simulink model "IID_nms_2Dmodel_for"  (R2016b)
settings: Solver=ode15s  StartTime=0.0  StopTime=t_end  FixedStep=1e-3  MaxStep=ts_max  RelTol=1e-3  AbsTol=1e-4  EnableMultiTasking=on
InitFcn:
  | IID_runScripts;
values from neighbouring files (symbols this model uses):
  D12_F = 0.16    [IID_nms_MechInit.m]    (also in nms_MechInit.m)
  D12_S = L_S    (= 0.5)    [IID_nms_MechInit.m]    (also in nms_MechInit.m = 0.46)
  D12_T = L_T    (= 0.5)    [IID_nms_MechInit.m]    (also in nms_MechInit.m = 0.46)
  D13_F = 0.20    (= 0.2)    [IID_nms_MechInit.m]    (also in nms_MechInit.m)
  D1G_F = 0.14    [IID_nms_MechInit.m]    (also in nms_MechInit.m)
  D1G_HAT = 0.35    [IID_nms_MechInit.m]    (also in nms_MechInit.m)
  D1G_S = 0.3    [IID_nms_MechInit.m]    (also in nms_MechInit.m = 0.28)
  D1G_T = 0.3    [IID_nms_MechInit.m]    (also in nms_MechInit.m = 0.28)
  DeltaThRef = 5e-3    (= 0.005)    [IID_nms_MechInit.m]    (also in nms_MechInit.m)
  Dist_On = 1    [IID_setDistPar.m]    (also in setDistPar.m)
  Dist_PDur = 0.15    [IID_setDistPar.m]    (also in setDistPar.m)
  Dist_StartTime = 15    [IID_setDistPar.m]    (also in setDistPar.m)
  Dist_xyzHAT_sag_PH = 0    [IID_setDistPar.m]    (also in setDistPar.m)
  In_F = 0.005    [IID_nms_MechInit.m]    (also in nms_MechInit.m)
  In_HAT = 3    [IID_nms_MechInit.m]    (also in nms_MechInit.m = 2.5)
  In_S = 0.05    [IID_nms_MechInit.m]    (also in nms_MechInit.m)
  In_T = 0.15    [IID_nms_MechInit.m]    (also in nms_MechInit.m)
  k_gx = (2*(m_F+m_S+m_T)+m_HAT)*g/0.1    (= 7848)    [IID_nms_MechInit.m]
  k_gy = (2*(m_F+m_S+m_T)+m_HAT)*g/0.01    (= 78480)    [IID_nms_MechInit.m]
  k_pressure = m_HAT * 9.81 / DeltaThRef    (= 104967)    [IID_nms_MechInit.m]    (also in nms_MechInit.m)
  m_F = 1.25    [IID_nms_MechInit.m]    (also in nms_MechInit.m)
  m_HAT = 53.5    [IID_nms_MechInit.m]    (also in nms_MechInit.m)
  m_S = 3.5    [IID_nms_MechInit.m]    (also in nms_MechInit.m)
  m_T = 8.5    [IID_nms_MechInit.m]    (also in nms_MechInit.m)
  m_Total = m_F*2+m_S*2+m_T*2+m_HAT    (= 80)    [IID_nms_MechInit.m]    (also in nms_MechInit.m)
  MidDelay = 0.010    (= 0.01)    [IID_setCtrlPar.m]    (also in nms_MechInit.m = 0.005)
  mu_slide = 0.8    [IID_nms_MechInit.m]    (also in nms_MechInit.m)
  mu_stick = 0.9    [IID_nms_MechInit.m]    (also in nms_MechInit.m)
  N = 1.5    [IID_nms_MechInit.m]    (also in cmaes_parfor.m = size(x,1); nms_MechInit.m)
  s = x(1:N-1,:).^2 + x(2:N,:).^2    [cmaes_parfor.m]
  ThPos = 4/5    (= 0.8)    [IID_nms_MechInit.m]    (also in nms_MechInit.m)
  v_gx_max = 0.03    [IID_nms_MechInit.m]
  v_gy_max = 0.03    [IID_nms_MechInit.m]
  v_max_pressure = 0.5    [IID_nms_MechInit.m]    (also in nms_MechInit.m)
  vLimit = 0.01    [IID_nms_MechInit.m]    (also in nms_MechInit.m)
undefined symbols (not defined in the file or in its folder): sgn
libraries: mblibv1 x71, cpg_lib x23, simulink x21, simulink_extras x6
(part 2 of 3)

== system IID_nms_2Dmodel_for/Signals NMC Left7 ==
  Mux : Mux  Inputs=7
  signals : Outport
  wires:
  Mux/1 -> signals/1
  [LEnergyVAS] -> Mux/2
  [LEnergyHFL] -> Mux/1
  [LEnergyTA] -> Mux/3
  [LEnergySOL] -> Mux/4
  [LEnergyHAM] -> Mux/6
  [LEnergyGAS] -> Mux/5
  [LEnergyGLU] -> Mux/7

== system IID_nms_2Dmodel_for/Signals NMC Right3 ==
  Mux : Mux
  signals : Outport
  wires:
  Mux/1 -> signals/1
  [RM34] -> Mux/1
  [RM23] -> Mux/3
  [RM12] -> Mux/4
  [RM34R] -> Mux/2

== system IID_nms_2Dmodel_for/etc ==
  note: Fall detection
      | (stop simulation)
  Abs3 : Abs
  Compare To Constant2 : simulink/Logic and Bit Operations/Compare To Constant  relop=>  const=60*pi/180  OutDataTypeStr=boolean
  Stop Simulation : Stop
  wires:
  Compare To Constant2/1 -> Stop Simulation/1
  Abs3/1 -> Compare To Constant2/1
  [theta] -> Abs3/1

== system IID_nms_2Dmodel_for/Body Mechanics Layer/Left Force Plate ==
  "GRF_Ball [N N] " : Inport
  GRF_Heel [N N] : Inport  Port=2
  Enable : EnablePort  StatesWhenEnabling=reset
  Fcn : Fcn  Expr=u(1)/(u(2)+eps)
  Mux : Mux  Inputs=3
  Mux1 : Mux  Inputs=2
  Selector : Selector  InputPortWidth=2  IndexOptions=Index vector (dialog)  Indices=2  OutputSizes=1
  Selector1 : Selector  InputPortWidth=2  IndexOptions=Index vector (dialog)  Indices=2  OutputSizes=1
  Sum1 : Sum
  GRFs : Outport  OutputWhenDisabled=reset  InitialOutput=0
  COP : Outport  Port=2  OutputWhenDisabled=reset  InitialOutput=0
  wires:
  Selector/1 -> Mux1/2
  Selector1/1 -> Mux1/1
  "GRF_Ball [N N] "/1 -> Sum1/1, Mux/1, Selector1/1
  GRF_Heel [N N]/1 -> Sum1/2, Mux/3
  Sum1/1 -> Mux/2, Selector/1
  Mux/1 -> GRFs/1
  Mux1/1 -> Fcn/1
  Fcn/1 -> COP/1

== system IID_nms_2Dmodel_for/Body Mechanics Layer/Left Leg Load ==
  dxThigh [m] : Inport
  FB Gain1 : Gain  Gain=1/DeltaThRef  SaturateOnIntegerOverflow=on  OutDataTypeStr=Inherit: Same as input  ParamDataTypeStr=Inherit: Same as input
  Saturation11 : Saturate  UpperLimit=inf  LowerLimit=0  ZeroCross=off
  smooth2 : TransferFcn  Denominator=[0.02 1]
  LLoad [F] : Outport
  wires:
  dxThigh [m]/1 -> smooth2/1
  FB Gain1/1 -> LLoad [F]/1
  smooth2/1 -> Saturation11/1
  Saturation11/1 -> FB Gain1/1

== system IID_nms_2Dmodel_for/Body Mechanics Layer/Left Thigh Sensor Sheet ==
  note: Inner Segment Pressure Sheet
  Gain3 : Gain  Gain=k_pressure
  Gain4 : Gain  Gain=1/v_max_pressure
  Inner Thigh Shift Joint : mblibv1/Joints/Prismatic  LConnTagsString=__newl0|SA1|SA2  RConnTagsString=__newr0|SA1  UpdateFromCAD=off  NumSAPorts=3  CutJoint=off  MarkAsCut=off  Primitives=prismatic  PrimitiveProps=P1$WORLD$[1 0 0]$prismatic  DialogClass=JointBlock  P1Axis=[1 0 0]
  Left Thigh Sensor Sheet IC : mblibv1/Sensors &  Actuators/Joint Initial Condition  UpdateFromCAD=off  LeftPortType=blob  RightPortType=blob  PhysicalDomain=mechanical  DialogClass=InitialConditionBlock  InitialConditions=P1$true$0$m$rad$0$m/s$rad/s#P2$false$0$m$rad$0$m/s$rad/s#P3$false$0$m$rad$0$m/s$rad/s#R1$false$0$m$rad$0$m/s$rad/s#R2$false$0$m$rad$0$m/s$rad/s#R3$false$0$m$rad$0$m/s$rad/s#S$false$0$m$rad$0$m/s$rad/s  P1PIC=0  P1VIC=0  P2PIC=0  P2VIC=0  P3PIC=0  P3VIC=0  R1PIC=0  R1VIC=0  R2PIC=0  R2VIC=0  R3PIC=0  R3VIC=0  SPIC=0  SVIC=0
  Mux1 : Mux  Inputs=2
  Pressure Sheet Reaction Force : Fcn  Expr=-u(1) * (1+sgn(u(1))*u(2))
  Thigh Actuator : mblibv1/Sensors &  Actuators/Joint Actuator  UpdateFromCAD=off  PhysicalDomain=Mechanical  PortType=blob  ActuationStyle=Force  AngleUnits=deg  ArcVelocityUnits=deg/s  ArcAccelerationUnits=deg/s^2  CoordPositionUnits=m  VelocityUnits=m/s  AccelerationUnits=m/s^2  ForceUnits=N  TorqueUnits=N-m  ActiveIO=on  Width=1  DialogClass=MechanicalActuatorBlock  Primitive=P1  ReferenceFrame=Absolute (INERTIAL)
  Thigh Sensor : mblibv1/Sensors &  Actuators/Joint Sensor  UpdateFromCAD=off  PhysicalDomain=Mechanical  PortType=blob  Muxed=off  Pose=off  Angle=on  AngleUnits=deg  ArcVelocity=off  ArcVelocityUnits=deg/s  ArcAcceleration=off  ArcAccelerationUnits=deg/s^2  CoordPosition=on  CoordPositionUnits=m  Velocity=on  VelocityUnits=m/s  Acceleration=off  AccelerationUnits=m/s^2  Quaternion=on  QuaternionDT=off  QuaternionDDT=off  QuaternionUnits=off  OutputVector=[ 1 1 ]  ActiveIO=on  Width=2  DialogClass=MechanicalSensorBlock  Primitive=P1  Force=off  ForceUnits=N  Torque=off  TorqueUnits=N-m  ReferenceFrame=Absolute (INERTIAL)  ReactionSensedSide=Base  ReactionReferenceFrame=Absolute (World)  ReactionForce=off  ReactionForceUnits=N  ReactionMoment=off  ReactionMomentUnits=N-m
  B : PMIOPort  Tag=PMCPort  Port=1  Side=Left
  F : PMIOPort  Tag=PMCPort  Port=2  Side=Right
  dx : Outport
  wires:
  Thigh Sensor/1 -> Gain3/1, dx/1
  Thigh Sensor/2 -> Gain4/1
  Mux1/1 -> Pressure Sheet Reaction Force/1
  Gain3/1 -> Mux1/1
  Gain4/1 -> Mux1/2
  Pressure Sheet Reaction Force/1 -> Thigh Actuator/1
  connections:
  B/RConn1 -- Inner Thigh Shift Joint/LConn1
  F/RConn1 -- Inner Thigh Shift Joint/RConn1
  Thigh Sensor/LConn1 -- Inner Thigh Shift Joint/LConn2
  Inner Thigh Shift Joint/RConn2 -- Thigh Actuator/RConn1
  Left Thigh Sensor Sheet IC/RConn1 -- Inner Thigh Shift Joint/LConn3

== system IID_nms_2Dmodel_for/Body Mechanics Layer/RLBall Cnt1 ==
  note: 3D Ground Interaction Model
  Dist_sag : Inport
  Body Actuator : mblibv1/Sensors &  Actuators/Body Actuator  UpdateFromCAD=off  PhysicalDomain=Mechanical  PortType=blob  ActuationStyle=Force  AngleUnits=deg  ArcVelocityUnits=deg/s  ArcAccelerationUnits=deg/s^2  CoordPositionUnits=m  VelocityUnits=m/s  AccelerationUnits=m/s^2  ForceUnits=N  TorqueUnits=N*m  ActiveIO=on  Width=3  DialogClass=MechanicalActuatorBlock  ReferenceFrame=Local (Body CS)  Angle=off  CoordPosition=on  Force=on  Torque=off
  Constant : Constant  Value=0
  Gain : Gain  Gain=-1
  Mechanical Branching Bar : mblibv1/Utilities/Mechanical Branching Bar  LConnTagsString=_newl0  RConnTagsString=SA0|SA1  UpdateFromCAD=off  DialogClass=MechanicalBranchingBarBlock  NumSAPorts=2
  Mux : Mux  Inputs=3
  Product : Product
  Product1 : Product
  Right Heel Sensor5 : mblibv1/Sensors &  Actuators/Body Sensor  UpdateFromCAD=off  PhysicalDomain=Mechanical  PortType=blob  Muxed=off  Pose=on  Angle=on  AngleUnits=deg  ArcVelocity=off  ArcVelocityUnits=deg/s  ArcAcceleration=off  ArcAccelerationUnits=deg/s^2  CoordPosition=on  CoordPositionUnits=m  Velocity=off  VelocityUnits=m/s  Acceleration=off  AccelerationUnits=m/s^2  Quaternion=on  QuaternionDT=off  QuaternionDDT=off  QuaternionUnits=off  OutputVector=[ 3 3 ]  ActiveIO=on  Width=12  DialogClass=MechanicalSensorBlock  ReferenceFrame=Absolute (World)
  Trigonometric Function : Trigonometry  Operator=cos
  Trigonometric Function1 : Trigonometry
  F : PMIOPort  Port=1  Side=Left
  Pos : Outport
  Rot : Outport  Port=2
  wires:
  Right Heel Sensor5/1 -> Pos/1  "pos"
  Mux/1 -> Body Actuator/1
  Constant/1 -> Mux/3
  Right Heel Sensor5/2 -> Rot/1
  [theta] -> Trigonometric Function/1, Trigonometric Function1/1
  Dist_sag/1 -> Product1/2, Product/2
  Trigonometric Function/1 -> Product/1
  Product/1 -> Gain/1
  Gain/1 -> Mux/2
  Trigonometric Function1/1 -> Product1/1
  Product1/1 -> Mux/1
  connections:
  F/RConn1 -- Mechanical Branching Bar/LConn1
  Mechanical Branching Bar/RConn2 -- Body Actuator/RConn1
  Mechanical Branching Bar/RConn1 -- Right Heel Sensor5/LConn1

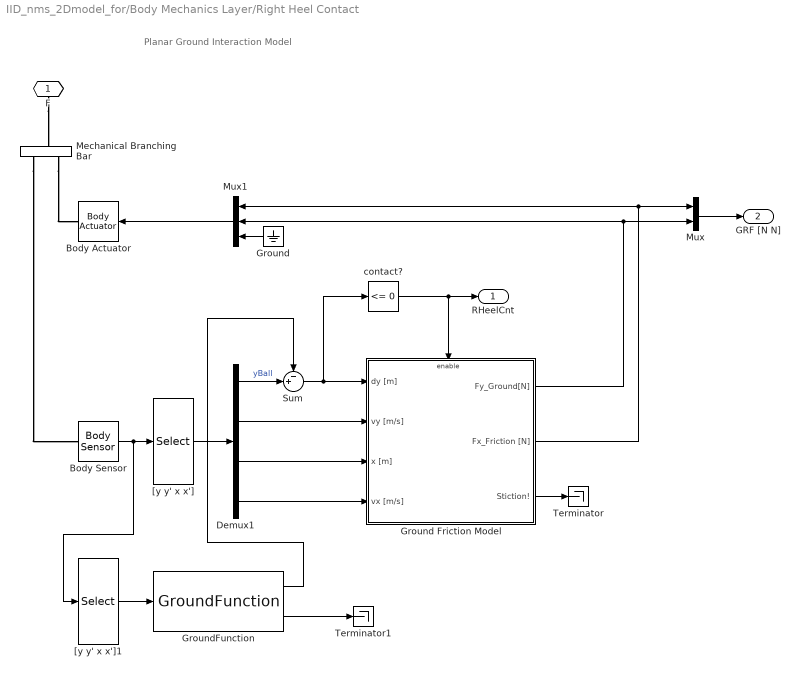
== system IID_nms_2Dmodel_for/Body Mechanics Layer/Right Heel Contact ==
  note: Planar Ground Interaction Model
  Body Actuator : mblibv1/Sensors &  Actuators/Body Actuator  UpdateFromCAD=off  PhysicalDomain=Mechanical  PortType=blob  ActuationStyle=Force  AngleUnits=deg  ArcVelocityUnits=deg/s  ArcAccelerationUnits=deg/s^2  CoordPositionUnits=m  VelocityUnits=m/s  AccelerationUnits=m/s^2  ForceUnits=N  TorqueUnits=N-m  ActiveIO=on  Width=3  DialogClass=MechanicalActuatorBlock  ReferenceFrame=Absolute (World)  Angle=off  CoordPosition=on  Force=on  Torque=off
  Body Sensor : mblibv1/Sensors &  Actuators/Body Sensor  UpdateFromCAD=off  PhysicalDomain=Mechanical  PortType=blob  Muxed=on  Pose=off  Angle=on  AngleUnits=deg  ArcVelocity=off  ArcVelocityUnits=deg/s  ArcAcceleration=off  ArcAccelerationUnits=deg/s^2  CoordPosition=on  CoordPositionUnits=m  Velocity=on  VelocityUnits=m/s  Acceleration=off  AccelerationUnits=m/s^2  Quaternion=on  QuaternionDT=off  QuaternionDDT=off  QuaternionUnits=off  OutputVector=[ 3 3 ]  ActiveIO=on  Width=6  DialogClass=MechanicalSensorBlock  ReferenceFrame=Absolute (World)
  Demux1 : Demux
  Ground : Ground
  Ground Friction Model : Subsystem
  GroundFunction : cpg_lib/GroundFunction
  Mechanical Branching Bar : mblibv1/Utilities/Mechanical Branching Bar  LConnTagsString=_newl0  RConnTagsString=SA0|SA1  UpdateFromCAD=off  DialogClass=MechanicalBranchingBarBlock  NumSAPorts=2
  Mux : Mux  Inputs=2
  Mux1 : Mux  Inputs=3
  Sum : Sum  Inputs=-+|
  Terminator : Terminator
  Terminator1 : Terminator
  "[y y' x x']" : Selector  InputPortWidth=6  IndexOptions=Index vector (dialog)  Indices=[2 5 1 4]  OutputSizes=1
  "[y y' x x']1" : Selector  InputPortWidth=6  IndexOptions=Index vector (dialog)  Indices=[1 2 3]  OutputSizes=1
  contact? : simulink/Logic and Bit Operations/Compare To Zero  relop=<=  OutDataTypeStr=boolean
  F : PMIOPort  Port=1  Side=Left
  RHeelCnt : Outport
  GRF [N N] : Outport  Port=2
  wires:
  Ground Friction Model/3(Stiction!) -> Terminator/1
  Ground Friction Model/2(Fx_Friction [N]) -> Mux/1, Mux1/1
  Ground Friction Model/1(Fy_Ground[N]) -> Mux/2, Mux1/2
  contact?/1 -> Ground Friction Model/Enable, RHeelCnt/1
  Demux1/4 -> Ground Friction Model/4(vx [m/s])
  Demux1/3 -> Ground Friction Model/3(x [m])
  Demux1/2 -> Ground Friction Model/2(vy [m/s])
  Mux/1 -> GRF [N N]/1
  GroundFunction/1 -> Sum/1
  Demux1/1 -> Sum/2  "yBall"
  Sum/1 -> Ground Friction Model/1(dy [m]), contact?/1
  Body Sensor/1 -> "[y y' x x']1"/1, "[y y' x x']"/1
  "[y y' x x']"/1 -> Demux1/1
  Mux1/1 -> Body Actuator/1
  Ground/1 -> Mux1/3
  "[y y' x x']1"/1 -> GroundFunction/1
  GroundFunction/2 -> Terminator1/1
  connections:
  F/RConn1 -- Mechanical Branching Bar/LConn1
  Mechanical Branching Bar/RConn1 -- Body Sensor/LConn1
  Mechanical Branching Bar/RConn2 -- Body Actuator/RConn1

== system IID_nms_2Dmodel_for/Body Mechanics Layer/Right Heel Contact1 ==
  note: Planar Ground Interaction Model
  Body Actuator : mblibv1/Sensors &  Actuators/Body Actuator  UpdateFromCAD=off  PhysicalDomain=Mechanical  PortType=blob  ActuationStyle=Force  AngleUnits=deg  ArcVelocityUnits=deg/s  ArcAccelerationUnits=deg/s^2  CoordPositionUnits=m  VelocityUnits=m/s  AccelerationUnits=m/s^2  ForceUnits=N  TorqueUnits=N-m  ActiveIO=on  Width=3  DialogClass=MechanicalActuatorBlock  ReferenceFrame=Absolute (World)  Angle=off  CoordPosition=on  Force=on  Torque=off
  Body Sensor : mblibv1/Sensors &  Actuators/Body Sensor  UpdateFromCAD=off  PhysicalDomain=Mechanical  PortType=blob  Muxed=on  Pose=off  Angle=on  AngleUnits=deg  ArcVelocity=off  ArcVelocityUnits=deg/s  ArcAcceleration=off  ArcAccelerationUnits=deg/s^2  CoordPosition=on  CoordPositionUnits=m  Velocity=on  VelocityUnits=m/s  Acceleration=off  AccelerationUnits=m/s^2  Quaternion=on  QuaternionDT=off  QuaternionDDT=off  QuaternionUnits=off  OutputVector=[ 3 3 ]  ActiveIO=on  Width=6  DialogClass=MechanicalSensorBlock  ReferenceFrame=Absolute (World)
  Demux1 : Demux
  Ground : Ground
  Ground Friction Model : Subsystem
  GroundFunction : cpg_lib/GroundFunction
  Mechanical Branching Bar : mblibv1/Utilities/Mechanical Branching Bar  LConnTagsString=_newl0  RConnTagsString=SA0|SA1  UpdateFromCAD=off  DialogClass=MechanicalBranchingBarBlock  NumSAPorts=2
  Mux : Mux  Inputs=2
  Mux1 : Mux  Inputs=3
  Sum : Sum  Inputs=-+|
  Terminator : Terminator
  Terminator1 : Terminator
  "[y y' x x']" : Selector  InputPortWidth=6  IndexOptions=Index vector (dialog)  Indices=[2 5 1 4]  OutputSizes=1
  "[y y' x x']1" : Selector  InputPortWidth=6  IndexOptions=Index vector (dialog)  Indices=[1 2 3]  OutputSizes=1
  contact? : simulink/Logic and Bit Operations/Compare To Zero  relop=<=  OutDataTypeStr=boolean
  F : PMIOPort  Port=1  Side=Left
  RHeelCnt : Outport
  GRF [N N] : Outport  Port=2
  wires:
  GroundFunction/2 -> Terminator1/1
  "[y y' x x']1"/1 -> GroundFunction/1
  Ground/1 -> Mux1/3
  Mux1/1 -> Body Actuator/1
  "[y y' x x']"/1 -> Demux1/1
  Body Sensor/1 -> "[y y' x x']"/1, "[y y' x x']1"/1
  Sum/1 -> contact?/1, Ground Friction Model/1(dy [m])
  Demux1/1 -> Sum/2  "yBall"
  GroundFunction/1 -> Sum/1
  Mux/1 -> GRF [N N]/1
  Demux1/2 -> Ground Friction Model/2(vy [m/s])
  Demux1/3 -> Ground Friction Model/3(x [m])
  Demux1/4 -> Ground Friction Model/4(vx [m/s])
  contact?/1 -> RHeelCnt/1, Ground Friction Model/Enable
  Ground Friction Model/1(Fy_Ground[N]) -> Mux1/2, Mux/2
  Ground Friction Model/2(Fx_Friction [N]) -> Mux1/1, Mux/1
  Ground Friction Model/3(Stiction!) -> Terminator/1
  connections:
  Mechanical Branching Bar/RConn2 -- Body Actuator/RConn1
  Mechanical Branching Bar/RConn1 -- Body Sensor/LConn1
  F/RConn1 -- Mechanical Branching Bar/LConn1

== system IID_nms_2Dmodel_for/Body Mechanics Layer/Right Heel Contact2 ==
  note: Planar Ground Interaction Model
  Body Actuator : mblibv1/Sensors &  Actuators/Body Actuator  UpdateFromCAD=off  PhysicalDomain=Mechanical  PortType=blob  ActuationStyle=Force  AngleUnits=deg  ArcVelocityUnits=deg/s  ArcAccelerationUnits=deg/s^2  CoordPositionUnits=m  VelocityUnits=m/s  AccelerationUnits=m/s^2  ForceUnits=N  TorqueUnits=N-m  ActiveIO=on  Width=3  DialogClass=MechanicalActuatorBlock  ReferenceFrame=Absolute (World)  Angle=off  CoordPosition=on  Force=on  Torque=off
  Body Sensor : mblibv1/Sensors &  Actuators/Body Sensor  UpdateFromCAD=off  PhysicalDomain=Mechanical  PortType=blob  Muxed=on  Pose=off  Angle=on  AngleUnits=deg  ArcVelocity=off  ArcVelocityUnits=deg/s  ArcAcceleration=off  ArcAccelerationUnits=deg/s^2  CoordPosition=on  CoordPositionUnits=m  Velocity=on  VelocityUnits=m/s  Acceleration=off  AccelerationUnits=m/s^2  Quaternion=on  QuaternionDT=off  QuaternionDDT=off  QuaternionUnits=off  OutputVector=[ 3 3 ]  ActiveIO=on  Width=6  DialogClass=MechanicalSensorBlock  ReferenceFrame=Absolute (World)
  Demux1 : Demux
  Ground : Ground
  Ground Friction Model : Subsystem
  GroundFunction : cpg_lib/GroundFunction
  Mechanical Branching Bar : mblibv1/Utilities/Mechanical Branching Bar  LConnTagsString=_newl0  RConnTagsString=SA0|SA1  UpdateFromCAD=off  DialogClass=MechanicalBranchingBarBlock  NumSAPorts=2
  Mux : Mux  Inputs=2
  Mux1 : Mux  Inputs=3
  Sum : Sum  Inputs=-+|
  Terminator : Terminator
  Terminator1 : Terminator
  "[y y' x x']" : Selector  InputPortWidth=6  IndexOptions=Index vector (dialog)  Indices=[2 5 1 4]  OutputSizes=1
  "[y y' x x']1" : Selector  InputPortWidth=6  IndexOptions=Index vector (dialog)  Indices=[1 2 3]  OutputSizes=1
  contact? : simulink/Logic and Bit Operations/Compare To Zero  relop=<=  OutDataTypeStr=boolean
  F : PMIOPort  Port=1  Side=Left
  RHeelCnt : Outport
  GRF [N N] : Outport  Port=2
  wires:
  Ground Friction Model/3(Stiction!) -> Terminator/1
  Ground Friction Model/2(Fx_Friction [N]) -> Mux/1, Mux1/1
  Ground Friction Model/1(Fy_Ground[N]) -> Mux/2, Mux1/2
  contact?/1 -> Ground Friction Model/Enable, RHeelCnt/1
  Demux1/4 -> Ground Friction Model/4(vx [m/s])
  Demux1/3 -> Ground Friction Model/3(x [m])
  Demux1/2 -> Ground Friction Model/2(vy [m/s])
  Mux/1 -> GRF [N N]/1
  GroundFunction/1 -> Sum/1
  Demux1/1 -> Sum/2  "yBall"
  Sum/1 -> Ground Friction Model/1(dy [m]), contact?/1
  Body Sensor/1 -> "[y y' x x']1"/1, "[y y' x x']"/1
  "[y y' x x']"/1 -> Demux1/1
  Mux1/1 -> Body Actuator/1
  Ground/1 -> Mux1/3
  "[y y' x x']1"/1 -> GroundFunction/1
  GroundFunction/2 -> Terminator1/1
  connections:
  F/RConn1 -- Mechanical Branching Bar/LConn1
  Mechanical Branching Bar/RConn1 -- Body Sensor/LConn1
  Mechanical Branching Bar/RConn2 -- Body Actuator/RConn1

== system IID_nms_2Dmodel_for/Body Mechanics Layer/Right Heel Contact3 ==
  note: Planar Ground Interaction Model
  Body Actuator : mblibv1/Sensors &  Actuators/Body Actuator  UpdateFromCAD=off  PhysicalDomain=Mechanical  PortType=blob  ActuationStyle=Force  AngleUnits=deg  ArcVelocityUnits=deg/s  ArcAccelerationUnits=deg/s^2  CoordPositionUnits=m  VelocityUnits=m/s  AccelerationUnits=m/s^2  ForceUnits=N  TorqueUnits=N-m  ActiveIO=on  Width=3  DialogClass=MechanicalActuatorBlock  ReferenceFrame=Absolute (World)  Angle=off  CoordPosition=on  Force=on  Torque=off
  Body Sensor : mblibv1/Sensors &  Actuators/Body Sensor  UpdateFromCAD=off  PhysicalDomain=Mechanical  PortType=blob  Muxed=on  Pose=off  Angle=on  AngleUnits=deg  ArcVelocity=off  ArcVelocityUnits=deg/s  ArcAcceleration=off  ArcAccelerationUnits=deg/s^2  CoordPosition=on  CoordPositionUnits=m  Velocity=on  VelocityUnits=m/s  Acceleration=off  AccelerationUnits=m/s^2  Quaternion=on  QuaternionDT=off  QuaternionDDT=off  QuaternionUnits=off  OutputVector=[ 3 3 ]  ActiveIO=on  Width=6  DialogClass=MechanicalSensorBlock  ReferenceFrame=Absolute (World)
  Demux1 : Demux
  Ground : Ground
  Ground Friction Model : Subsystem
  GroundFunction : cpg_lib/GroundFunction
  Mechanical Branching Bar : mblibv1/Utilities/Mechanical Branching Bar  LConnTagsString=_newl0  RConnTagsString=SA0|SA1  UpdateFromCAD=off  DialogClass=MechanicalBranchingBarBlock  NumSAPorts=2
  Mux : Mux  Inputs=2
  Mux1 : Mux  Inputs=3
  Sum : Sum  Inputs=-+|
  Terminator : Terminator
  Terminator1 : Terminator
  "[y y' x x']" : Selector  InputPortWidth=6  IndexOptions=Index vector (dialog)  Indices=[2 5 1 4]  OutputSizes=1
  "[y y' x x']1" : Selector  InputPortWidth=6  IndexOptions=Index vector (dialog)  Indices=[1 2 3]  OutputSizes=1
  contact? : simulink/Logic and Bit Operations/Compare To Zero  relop=<=  OutDataTypeStr=boolean
  F : PMIOPort  Port=1  Side=Left
  RHeelCnt : Outport
  GRF [N N] : Outport  Port=2
  wires:
  GroundFunction/2 -> Terminator1/1
  "[y y' x x']1"/1 -> GroundFunction/1
  Ground/1 -> Mux1/3
  Mux1/1 -> Body Actuator/1
  "[y y' x x']"/1 -> Demux1/1
  Body Sensor/1 -> "[y y' x x']"/1, "[y y' x x']1"/1
  Sum/1 -> contact?/1, Ground Friction Model/1(dy [m])
  Demux1/1 -> Sum/2  "yBall"
  GroundFunction/1 -> Sum/1
  Mux/1 -> GRF [N N]/1
  Demux1/2 -> Ground Friction Model/2(vy [m/s])
  Demux1/3 -> Ground Friction Model/3(x [m])
  Demux1/4 -> Ground Friction Model/4(vx [m/s])
  contact?/1 -> RHeelCnt/1, Ground Friction Model/Enable
  Ground Friction Model/1(Fy_Ground[N]) -> Mux1/2, Mux/2
  Ground Friction Model/2(Fx_Friction [N]) -> Mux1/1, Mux/1
  Ground Friction Model/3(Stiction!) -> Terminator/1
  connections:
  Mechanical Branching Bar/RConn2 -- Body Actuator/RConn1
  Mechanical Branching Bar/RConn1 -- Body Sensor/LConn1
  F/RConn1 -- Mechanical Branching Bar/LConn1

== system IID_nms_2Dmodel_for/Body Mechanics Layer/Right Force Plate ==
  "GRF_Ball [N N] " : Inport
  GRF_Heel [N N] : Inport  Port=2
  Enable : EnablePort  StatesWhenEnabling=reset
  Fcn : Fcn  Expr=u(1)/(u(2)+eps)
  Mux : Mux  Inputs=3
  Mux1 : Mux  Inputs=2
  Selector : Selector  InputPortWidth=2  IndexOptions=Index vector (dialog)  Indices=2  OutputSizes=1
  Selector1 : Selector  InputPortWidth=2  IndexOptions=Index vector (dialog)  Indices=2  OutputSizes=1
  Sum1 : Sum
  GRFs : Outport  OutputWhenDisabled=reset  InitialOutput=0
  COP : Outport  Port=2  OutputWhenDisabled=reset  InitialOutput=0
  wires:
  Selector/1 -> Mux1/2
  Selector1/1 -> Mux1/1
  "GRF_Ball [N N] "/1 -> Sum1/1, Mux/1, Selector1/1
  GRF_Heel [N N]/1 -> Sum1/2, Mux/3
  Sum1/1 -> Mux/2, Selector/1
  Mux/1 -> GRFs/1
  Mux1/1 -> Fcn/1
  Fcn/1 -> COP/1

== system IID_nms_2Dmodel_for/Body Mechanics Layer/Right Leg Load ==
  dxThigh [m] : Inport
  FB Gain1 : Gain  Gain=1/DeltaThRef  SaturateOnIntegerOverflow=on  OutDataTypeStr=Inherit: Same as input  ParamDataTypeStr=Inherit: Same as input
  Saturation11 : Saturate  UpperLimit=inf  LowerLimit=0  ZeroCross=off
  smooth2 : TransferFcn  Denominator=[0.02 1]
  LLoad [F] : Outport
  wires:
  dxThigh [m]/1 -> smooth2/1
  FB Gain1/1 -> LLoad [F]/1
  smooth2/1 -> Saturation11/1
  Saturation11/1 -> FB Gain1/1

== system IID_nms_2Dmodel_for/Body Mechanics Layer/Right Thigh Sensor Sheet ==
  note: Inner Segment Pressure Sheet
  Gain3 : Gain  Gain=k_pressure
  Gain4 : Gain  Gain=1/v_max_pressure
  Inner Thigh Shift Joint : mblibv1/Joints/Prismatic  LConnTagsString=__newl0|SA1|SA2  RConnTagsString=__newr0|SA1  UpdateFromCAD=off  NumSAPorts=3  CutJoint=off  MarkAsCut=off  Primitives=prismatic  PrimitiveProps=P1$WORLD$[1 0 0]$prismatic  DialogClass=JointBlock  P1Axis=[1 0 0]
  Mux1 : Mux  Inputs=2
  Pressure Sheet Reaction Force : Fcn  Expr=-u(1) * (1+sgn(u(1))*u(2))
  Right Thigh Sensor Sheet IC : mblibv1/Sensors &  Actuators/Joint Initial Condition  UpdateFromCAD=off  LeftPortType=blob  RightPortType=blob  PhysicalDomain=mechanical  DialogClass=InitialConditionBlock  InitialConditions=P1$true$0$m$rad$0$m/s$rad/s#P2$false$0$m$rad$0$m/s$rad/s#P3$false$0$m$rad$0$m/s$rad/s#R1$false$0$m$rad$0$m/s$rad/s#R2$false$0$m$rad$0$m/s$rad/s#R3$false$0$m$rad$0$m/s$rad/s#S$false$0$m$rad$0$m/s$rad/s  P1PIC=0  P1VIC=0  P2PIC=0  P2VIC=0  P3PIC=0  P3VIC=0  R1PIC=0  R1VIC=0  R2PIC=0  R2VIC=0  R3PIC=0  R3VIC=0  SPIC=0  SVIC=0
  Thigh Actuator : mblibv1/Sensors &  Actuators/Joint Actuator  UpdateFromCAD=off  PhysicalDomain=Mechanical  PortType=blob  ActuationStyle=Force  AngleUnits=deg  ArcVelocityUnits=deg/s  ArcAccelerationUnits=deg/s^2  CoordPositionUnits=m  VelocityUnits=m/s  AccelerationUnits=m/s^2  ForceUnits=N  TorqueUnits=N-m  ActiveIO=on  Width=1  DialogClass=MechanicalActuatorBlock  Primitive=P1  ReferenceFrame=Absolute (INERTIAL)
  Thigh Sensor : mblibv1/Sensors &  Actuators/Joint Sensor  UpdateFromCAD=off  PhysicalDomain=Mechanical  PortType=blob  Muxed=off  Pose=off  Angle=on  AngleUnits=deg  ArcVelocity=off  ArcVelocityUnits=deg/s  ArcAcceleration=off  ArcAccelerationUnits=deg/s^2  CoordPosition=on  CoordPositionUnits=m  Velocity=on  VelocityUnits=m/s  Acceleration=off  AccelerationUnits=m/s^2  Quaternion=on  QuaternionDT=off  QuaternionDDT=off  QuaternionUnits=off  OutputVector=[ 1 1 ]  ActiveIO=on  Width=2  DialogClass=MechanicalSensorBlock  Primitive=P1  Force=off  ForceUnits=N  Torque=off  TorqueUnits=N-m  ReferenceFrame=Absolute (INERTIAL)  ReactionSensedSide=Base  ReactionReferenceFrame=Absolute (World)  ReactionForce=off  ReactionForceUnits=N  ReactionMoment=off  ReactionMomentUnits=N-m
  B : PMIOPort  Tag=PMCPort  Port=1  Side=Left
  F : PMIOPort  Tag=PMCPort  Port=2  Side=Right
  dx : Outport
  wires:
  Thigh Sensor/1 -> Gain3/1, dx/1
  Thigh Sensor/2 -> Gain4/1
  Mux1/1 -> Pressure Sheet Reaction Force/1
  Gain3/1 -> Mux1/1
  Gain4/1 -> Mux1/2
  Pressure Sheet Reaction Force/1 -> Thigh Actuator/1
  connections:
  B/RConn1 -- Inner Thigh Shift Joint/LConn1
  F/RConn1 -- Inner Thigh Shift Joint/RConn1
  Thigh Sensor/LConn1 -- Inner Thigh Shift Joint/LConn2
  Inner Thigh Shift Joint/RConn2 -- Thigh Actuator/RConn1
  Inner Thigh Shift Joint/LConn3 -- Right Thigh Sensor Sheet IC/RConn1

== system IID_nms_2Dmodel_for/Data Logging/Angles1 ==
  Constant : Constant  Value=zeros(2,1)
  Constant1 : Constant  Value=zeros(2,1)
  Mux : Mux  Inputs=8
  Angles : Outport
  wires:
  [Rphi12dphi12] -> Mux/8
  [Lphi34dphi34] -> Mux/1
  [Rphi23dphi23] -> Mux/7
  [Lphi23dphi23] -> Mux/3
  Constant1/1 -> Mux/6
  Constant/1 -> Mux/2
  [Lphi12dphi12] -> Mux/4
  [Rphi34dphi34] -> Mux/5
  Mux/1 -> Angles/1

== system IID_nms_2Dmodel_for/Data Logging/BodyInfo1 ==
  Angles : Inport
  Postitions : Inport  Port=2
  Loads : Inport  Port=3
  Mux1 : Mux  Inputs=3
  To File8 : ToFile  Filename=Records/BodyInfo
  wires:
  Loads/1 -> Mux1/3
  Postitions/1 -> Mux1/2
  Mux1/1 -> To File8/1
  Angles/1 -> Mux1/1

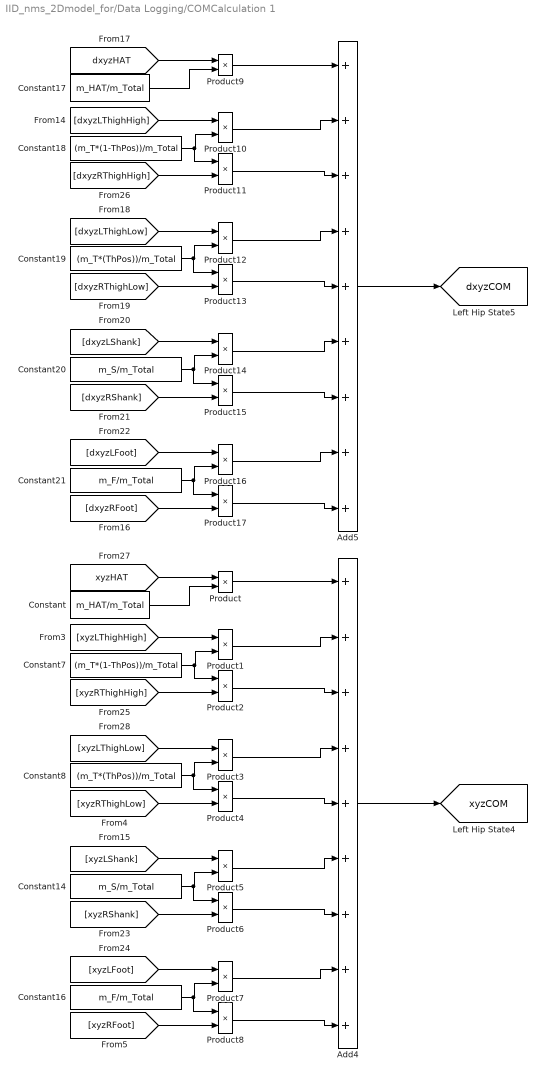
== system IID_nms_2Dmodel_for/Data Logging/COMCalculation 1 ==
  Add4 : Sum  Inputs=9
  Add5 : Sum  Inputs=9
  Constant : Constant  Value=m_HAT/m_Total
  Constant14 : Constant  Value=m_S/m_Total
  Constant16 : Constant  Value=m_F/m_Total
  Constant17 : Constant  Value=m_HAT/m_Total
  Constant18 : Constant  Value=(m_T*(1-ThPos))/m_Total
  Constant19 : Constant  Value=(m_T*(ThPos))/m_Total
  Constant20 : Constant  Value=m_S/m_Total
  Constant21 : Constant  Value=m_F/m_Total
  Constant7 : Constant  Value=(m_T*(1-ThPos))/m_Total
  Constant8 : Constant  Value=(m_T*(ThPos))/m_Total
  Product{,1..17} (18 alike) : Product
  tag scope: dxyzCOM=global, xyzCOM=global
  wires:
  [xyzRThighHigh] -> Product2/2
  [xyzRShank] -> Product6/2
  Constant/1 -> Product/2
  Constant20/1 -> Product14/2, Product15/1
  Product12/1 -> Add5/4
  [dxyzLShank] -> Product14/1
  [dxyzHAT] -> Product9/1
  Product10/1 -> Add5/2
  Constant8/1 -> Product3/2, Product4/1
  Product15/1 -> Add5/7
  Product16/1 -> Add5/8
  Product5/1 -> Add4/6
  Product7/1 -> Add4/8
  [dxyzRShank] -> Product15/2
  [xyzRThighLow] -> Product4/2
  Product1/1 -> Add4/2
  Product3/1 -> Add4/4
  Constant17/1 -> Product9/2
  Product9/1 -> Add5/1
  Product13/1 -> Add5/5
  Product17/1 -> Add5/9
  Product/1 -> Add4/1
  [xyzLThighLow] -> Product3/1
  Constant16/1 -> Product7/2, Product8/1
  [dxyzRFoot] -> Product17/2
  [xyzLFoot] -> Product7/1
  Constant19/1 -> Product13/1, Product12/2
  [xyzRFoot] -> Product8/2
  [dxyzRThighLow] -> Product13/2
  Product2/1 -> Add4/3
  Add4/1 -> [xyzCOM]
  Constant14/1 -> Product6/1, Product5/2
  [xyzLThighHigh] -> Product1/1
  Constant7/1 -> Product1/2, Product2/1
  [dxyzLFoot] -> Product16/1
  [xyzHAT] -> Product/1
  Constant21/1 -> Product17/1, Product16/2
  [dxyzLThighLow] -> Product12/1
  [dxyzRThighHigh] -> Product11/2
  Add5/1 -> [dxyzCOM]
  [xyzLShank] -> Product5/1
  Constant18/1 -> Product11/1, Product10/2
  Product14/1 -> Add5/6
  Product8/1 -> Add4/9
  Product11/1 -> Add5/3
  [dxyzLThighHigh] -> Product10/1
  Product6/1 -> Add4/7
  Product4/1 -> Add4/5

== system IID_nms_2Dmodel_for/Data Logging/Dist ==
  Dist : Outport
  wires:
  [xyzHAT_D_sag] -> Dist/1

== system IID_nms_2Dmodel_for/Data Logging/Disturbances ==
  Dist : Inport
  To File21 : ToFile  Filename=Records/Disturbance
  wires:
  Dist/1 -> To File21/1

== system IID_nms_2Dmodel_for/Data Logging/Joint Torques2 ==
  Target : Inport
  To File12 : ToFile  Filename=Records/TargetAngle
  wires:
  Target/1 -> To File12/1

== system IID_nms_2Dmodel_for/Data Logging/Joint TorquesPassive1 ==
  LTor : Inport
  RTor : Inport  Port=2
  To File12 : ToFile  Filename=Records/L_Tor_Passive
  To File9 : ToFile  Filename=Records/R_Tor_Passvie
  wires:
  RTor/1 -> To File9/1
  LTor/1 -> To File12/1

== system IID_nms_2Dmodel_for/Data Logging/Joint TorquesTotal1 ==
  LTor : Inport
  RTor : Inport  Port=2
  To File12 : ToFile  Filename=Records/L_Tor
  To File9 : ToFile  Filename=Records/R_Tor
  wires:
  LTor/1 -> To File12/1
  RTor/1 -> To File9/1

== system IID_nms_2Dmodel_for/Data Logging/Loads1 ==
  Mux : Mux  Inputs=2
  Loads : Outport
  wires:
  [LLLoad] -> Mux/2
  [RLLoad] -> Mux/1
  Mux/1 -> Loads/1

== system IID_nms_2Dmodel_for/Data Logging/M1 ==
  M11 : Inport
  To File2 : ToFile  Filename=Records/M11
  wires:
  M11/1 -> To File2/1

== system IID_nms_2Dmodel_for/Data Logging/Muscle Activation1 ==
  L_MA : Inport
  R_MA : Inport  Port=2
  To File1 : ToFile  Filename=Records/R_MA
  To File5 : ToFile  Filename=Records/L_MA
  wires:
  L_MA/1 -> To File5/1
  R_MA/1 -> To File1/1

== system IID_nms_2Dmodel_for/Data Logging/Muscle Power1 ==
  L_MA : Inport
  R_MA : Inport  Port=2
  To File1 : ToFile  Filename=Records/R_Power
  To File5 : ToFile  Filename=Records/L_Power
  wires:
  L_MA/1 -> To File5/1
  R_MA/1 -> To File1/1

== system IID_nms_2Dmodel_for/Data Logging/Positions1 ==
  Mux : Mux  Inputs=19
  Positions : Outport
  wires:
  [xyzRBall] -> Mux/19, Mux/18
  [xyzRHeel] -> Mux/17, Mux/16
  [xyzLBall] -> Mux/15, Mux/14
  [xyzLHeel] -> Mux/13, Mux/12
  [xyzTrunk] -> Mux/11
  [dxyzHAT] -> Mux/2
  [xyzHAT] -> Mux/1
  [dxyzRHip] -> Mux/10
  [xyzRHip] -> Mux/9
  [xyzLAnkle] -> Mux/3
  [xyzRKnee] -> Mux/8
  [dxyzLHip] -> Mux/6
  [xyzLHip] -> Mux/5
  [xyzLKnee] -> Mux/4
  [xyzRAnkle] -> Mux/7
  Mux/1 -> Positions/1

== system IID_nms_2Dmodel_for/Data Logging/Signals NMC Left1 ==
  Mux : Mux
  Target : Outport
  wires:
  Mux/1 -> Target/1
  [Lalpha_tgt] -> Mux/1
  [LhipR_tgt] -> Mux/3
  [RhipR_tgt] -> Mux/4
  [Ralpha_tgt] -> Mux/2

== system IID_nms_2Dmodel_for/Data Logging/Signals NMC Left10 ==
  Mux : Mux  Inputs=11
  signals : Outport
  wires:
  [LEnergyRF] -> Mux/2
  [LEnergyTA] -> Mux/4
  [LEnergyGAS] -> Mux/6
  [LEnergyHAM] -> Mux/8
  [LEnergyHAB] -> Mux/10
  [LEnergySOL] -> Mux/5
  [LEnergyHAD] -> Mux/11
  [LEnergyBFSH] -> Mux/7
  [LEnergyVAS] -> Mux/3
  [LEnergyGLU] -> Mux/9
  [LEnergyHFL] -> Mux/1
  Mux/1 -> signals/1

== system IID_nms_2Dmodel_for/Data Logging/Signals NMC Left2 ==
  Mux : Mux  Inputs=11
  signals : Outport
  wires:
  [LStimRF] -> Mux/2
  [LStimTA] -> Mux/4
  [LStimGAS] -> Mux/6
  [LStimHAM] -> Mux/8
  [LStimHAB] -> Mux/10
  [LStimSOL] -> Mux/5
  [LStimHAD] -> Mux/11
  [LStimBFSH] -> Mux/7
  [LStimVAS] -> Mux/3
  [LStimGLU] -> Mux/9
  [LStimHFL] -> Mux/1
  Mux/1 -> signals/1

== system IID_nms_2Dmodel_for/Data Logging/Signals NMC Left5 ==
  Mux : Mux
  signals : Outport
  wires:
  [LM34R] -> Mux/2
  [LM12] -> Mux/4
  [LM23] -> Mux/3
  [LM34] -> Mux/1
  Mux/1 -> signals/1

== system IID_nms_2Dmodel_for/Data Logging/Signals NMC Left8 ==
  Mux : Mux
  signals : Outport
  wires:
  Mux/1 -> signals/1
  [LHipStop] -> Mux/1
  [LKneeStop] -> Mux/3
  [LAnkleStop] -> Mux/4
  [LHipRStop] -> Mux/2

== system IID_nms_2Dmodel_for/Data Logging/Signals NMC Left9 ==
  Mux : Mux  Inputs=11
  signals : Outport
  wires:
  Mux/1 -> signals/1
  [REnergyHFL] -> Mux/1
  [REnergyGLU] -> Mux/9
  [REnergyVAS] -> Mux/3
  [REnergyBFSH] -> Mux/7
  [REnergyHAD] -> Mux/11
  [REnergySOL] -> Mux/5
  [REnergyHAB] -> Mux/10
  [REnergyHAM] -> Mux/8
  [REnergyGAS] -> Mux/6
  [REnergyTA] -> Mux/4
  [REnergyRF] -> Mux/2

== system IID_nms_2Dmodel_for/Data Logging/Signals NMC Right2 ==
  Mux : Mux
  signals : Outport
  wires:
  Mux/1 -> signals/1
  [RHipStop] -> Mux/1
  [RKneeStop] -> Mux/3
  [RAnkleStop] -> Mux/4
  [RHipStopR] -> Mux/2

== system IID_nms_2Dmodel_for/Data Logging/Signals NMC Right4 ==
  Mux : Mux  Inputs=11
  signals : Outport
  wires:
  Mux/1 -> signals/1
  [RStimHFL] -> Mux/1
  [RStimGLU] -> Mux/9
  [RStimVAS] -> Mux/3
  [RStimBFSH] -> Mux/7
  [RStimHAD] -> Mux/11
  [RStimSOL] -> Mux/5
  [RStimHAB] -> Mux/10
  [RStimHAM] -> Mux/8
  [RStimGAS] -> Mux/6
  [RStimTA] -> Mux/4
  [RStimRF] -> Mux/2

== system IID_nms_2Dmodel_for/Data Logging/Signals NMC Right5 ==
  Mux : Mux
  signals : Outport
  wires:
  [RM34R] -> Mux/2
  [RM12] -> Mux/4
  [RM23] -> Mux/3
  [RM34] -> Mux/1
  Mux/1 -> signals/1

== system IID_nms_2Dmodel_for/Data Logging/StanceInfo1 ==
  LStance : Inport
  RStance : Inport  Port=2
  Mux4 : Mux  Inputs=2
  To File4 : ToFile  Filename=Records/StanceSig
  wires:
  LStance/1 -> Mux4/1
  RStance/1 -> Mux4/2
  Mux4/1 -> To File4/1

== system IID_nms_2Dmodel_for/Data Logging/Subsystem1 ==
  RotTrunk : Inport
  To File8 : ToFile  Filename=Records/rotTrunk
  wires:
  RotTrunk/1 -> To File8/1

== system IID_nms_2Dmodel_for/Disturbances/Disturbances ==
  Dist : Inport
  Demux : Demux  Outputs=1
  tag scope: xyzHAT_D_sag=global
  wires:
  Demux/1 -> [xyzHAT_D_sag]
  Dist/1 -> Demux/1

== system IID_nms_2Dmodel_for/Disturbances/SampleAndHold ==
  Sample : Inport
  Value : Inport  Port=2
  IC=ic : Memory  LinearizeAsDelay=on
  Switch : Switch  Threshold=0.5  SaturateOnIntegerOverflow=on
  Out : Outport
  wires:
  Sample/1 -> Switch/2
  Switch/1 -> IC=ic/1, Out/1
  IC=ic/1 -> Switch/3
  Value/1 -> Switch/1

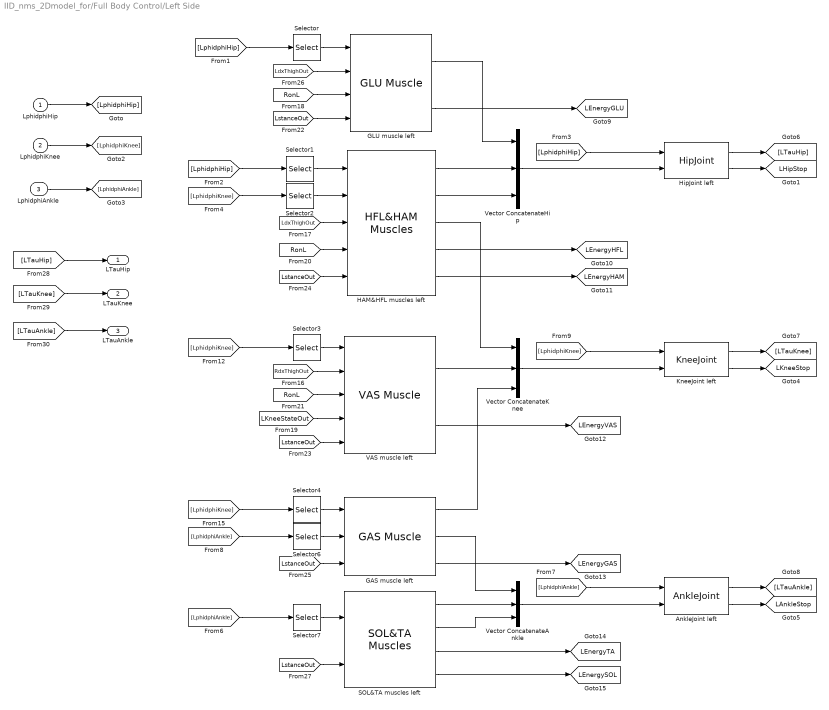
== system IID_nms_2Dmodel_for/Full Body Control/Left Side ==
  LphidphiHip : Inport
  LphidphiKnee : Inport  Port=2
  LphidphiAnkle : Inport  Port=3
  AnkleJoint left : cpg_lib/AnkleJoint
  GAS muscle left : cpg_lib/GAS Muscle
  GLU muscle left : cpg_lib/GLU Muscle
  HAM&HFL muscles left : cpg_lib/HFL&HAM Muscles
  HipJoint left : cpg_lib/HipJoint
  KneeJoint left : cpg_lib/KneeJoint
  SOL&TA muscles left : cpg_lib/SOL&TA Muscles
  Selector{,1..4,6..7} (7 alike) : Selector  InputPortWidth=2  IndexOptions=Index vector (dialog)  Indices=[1 ]  OutputSizes=1
  VAS muscle left : cpg_lib/VAS Muscle
  Vector ConcatenateAnkle : Concatenate  NumInputs=3
  Vector ConcatenateHip : Concatenate  NumInputs=3
  Vector ConcatenateKnee : Concatenate  NumInputs=3
  LTauHip : Outport
  LTauKnee : Outport  Port=2
  LTauAnkle : Outport  Port=3
  tag scope: LAnkleStop=global, LEnergyGAS=global, LEnergyGLU=global, LEnergyHAM=global, LEnergyHFL=global, LEnergySOL=global, LEnergyTA=global, LEnergyVAS=global, LHipStop=global, LKneeStop=global
  wires:
  GAS muscle left/2 -> Vector ConcatenateAnkle/1
  Vector ConcatenateHip/1 -> HipJoint left/2
  [LphidphiKnee] -> KneeJoint left/1
  Selector1/1 -> HAM&HFL muscles left/1
  Selector4/1 -> GAS muscle left/1
  [RdxThighOut] -> VAS muscle left/2
  SOL&TA muscles left/2 -> Vector ConcatenateAnkle/3
  Selector7/1 -> SOL&TA muscles left/1
  Vector ConcatenateAnkle/1 -> AnkleJoint left/2
  Vector ConcatenateKnee/1 -> KneeJoint left/2
  SOL&TA muscles left/1 -> Vector ConcatenateAnkle/2
  Selector3/1 -> VAS muscle left/1
  Selector6/1 -> GAS muscle left/2
  VAS muscle left/1 -> Vector ConcatenateKnee/2
  [LphidphiAnkle] -> AnkleJoint left/1
  GAS muscle left/1 -> Vector ConcatenateKnee/3
  HAM&HFL muscles left/1 -> Vector ConcatenateHip/2
  GLU muscle left/1 -> Vector ConcatenateHip/1
  [LstanceOut] -> HAM&HFL muscles left/5
  [RonL] -> VAS muscle left/3
  [LphidphiKnee] -> Selector3/1
  [LphidphiKnee] -> Selector4/1
  [RonL] -> HAM&HFL muscles left/4
  [LKneeStateOut] -> VAS muscle left/4
  HAM&HFL muscles left/3 -> Vector ConcatenateKnee/1
  Selector/1 -> GLU muscle left/1
  [LstanceOut] -> GAS muscle left/3
  [LphidphiAnkle] -> Selector7/1
  [LstanceOut] -> SOL&TA muscles left/2
  HAM&HFL muscles left/2 -> Vector ConcatenateHip/3
  Selector2/1 -> HAM&HFL muscles left/2
  [LphidphiAnkle] -> Selector6/1
  [LphidphiHip] -> Selector1/1
  [LstanceOut] -> VAS muscle left/5
  [LphidphiHip] -> Selector/1
  [LphidphiHip] -> HipJoint left/1
  [LphidphiKnee] -> Selector2/1
  HipJoint left/1 -> [LTauHip]
  KneeJoint left/1 -> [LTauKnee]
  AnkleJoint left/1 -> [LTauAnkle]
  [LdxThighOut] -> GLU muscle left/2
  [LstanceOut] -> GLU muscle left/4
  [RonL] -> GLU muscle left/3
  [LdxThighOut] -> HAM&HFL muscles left/3
  LphidphiHip/1 -> [LphidphiHip]
  LphidphiKnee/1 -> [LphidphiKnee]
  LphidphiAnkle/1 -> [LphidphiAnkle]
  [LTauHip] -> LTauHip/1
  [LTauKnee] -> LTauKnee/1
  [LTauAnkle] -> LTauAnkle/1
  HipJoint left/2 -> [LHipStop]
  KneeJoint left/2 -> [LKneeStop]
  AnkleJoint left/2 -> [LAnkleStop]
  GLU muscle left/2 -> [LEnergyGLU]
  HAM&HFL muscles left/4 -> [LEnergyHFL]
  HAM&HFL muscles left/5 -> [LEnergyHAM]
  VAS muscle left/2 -> [LEnergyVAS]
  GAS muscle left/3 -> [LEnergyGAS]
  SOL&TA muscles left/3 -> [LEnergyTA]
  SOL&TA muscles left/4 -> [LEnergySOL]

== system IID_nms_2Dmodel_for/Full Body Control/Main Control Goto ==
  EnableNMC_JointLimits : Inport
  tag scope: DisableNMC_JointLimits=global
  wires:
  EnableNMC_JointLimits/1 -> [DisableNMC_JointLimits]

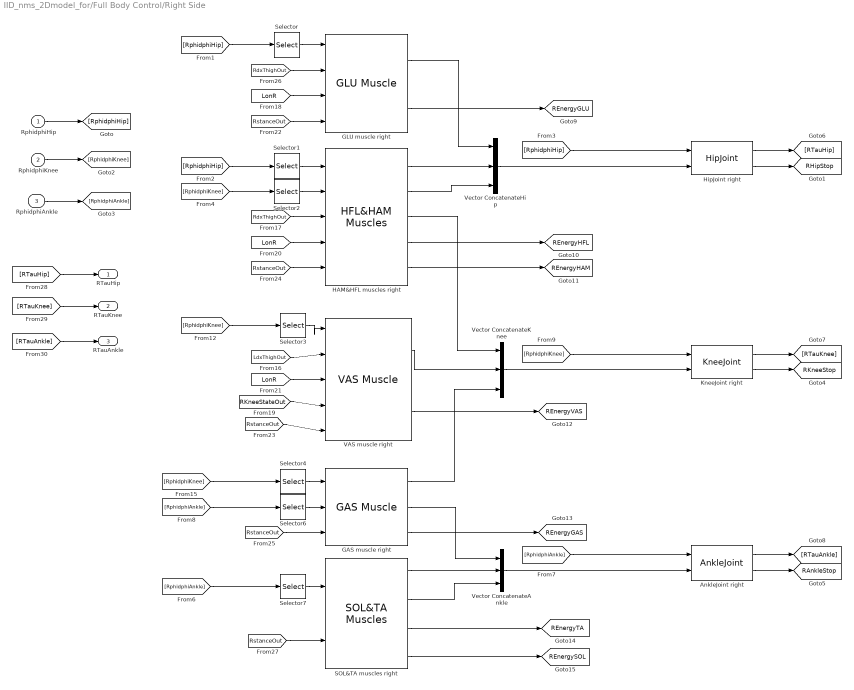
== system IID_nms_2Dmodel_for/Full Body Control/Right Side ==
  RphidphiHip : Inport
  RphidphiKnee : Inport  Port=2
  RphidphiAnkle : Inport  Port=3
  AnkleJoint right : cpg_lib/AnkleJoint
  GAS muscle right : cpg_lib/GAS Muscle
  GLU muscle right : cpg_lib/GLU Muscle
  HAM&HFL muscles right : cpg_lib/HFL&HAM Muscles
  HipJoint right : cpg_lib/HipJoint
  KneeJoint right : cpg_lib/KneeJoint
  SOL&TA muscles right : cpg_lib/SOL&TA Muscles
  Selector{,1..4,6..7} (7 alike) : Selector  InputPortWidth=2  IndexOptions=Index vector (dialog)  Indices=[1 ]  OutputSizes=1
  VAS muscle right : cpg_lib/VAS Muscle
  Vector ConcatenateAnkle : Concatenate  NumInputs=3
  Vector ConcatenateHip : Concatenate  NumInputs=3
  Vector ConcatenateKnee : Concatenate  NumInputs=3
  RTauHip : Outport
  RTauKnee : Outport  Port=2
  RTauAnkle : Outport  Port=3
  tag scope: RAnkleStop=global, REnergyGAS=global, REnergyGLU=global, REnergyHAM=global, REnergyHFL=global, REnergySOL=global, REnergyTA=global, REnergyVAS=global, RHipStop=global, RKneeStop=global
  wires:
  GAS muscle right/2 -> Vector ConcatenateAnkle/1
  Vector ConcatenateHip/1 -> HipJoint right/2
  [RphidphiKnee] -> KneeJoint right/1
  Selector1/1 -> HAM&HFL muscles right/1
  Selector4/1 -> GAS muscle right/1
  [LdxThighOut] -> VAS muscle right/2
  SOL&TA muscles right/2 -> Vector ConcatenateAnkle/3
  Selector7/1 -> SOL&TA muscles right/1
  Vector ConcatenateAnkle/1 -> AnkleJoint right/2
  Vector ConcatenateKnee/1 -> KneeJoint right/2
  SOL&TA muscles right/1 -> Vector ConcatenateAnkle/2
  Selector3/1 -> VAS muscle right/1
  Selector6/1 -> GAS muscle right/2
  VAS muscle right/1 -> Vector ConcatenateKnee/2
  [RphidphiAnkle] -> AnkleJoint right/1
  GAS muscle right/1 -> Vector ConcatenateKnee/3
  HAM&HFL muscles right/1 -> Vector ConcatenateHip/2
  GLU muscle right/1 -> Vector ConcatenateHip/1
  [LonR] -> VAS muscle right/3
  [RphidphiKnee] -> Selector3/1
  [RphidphiKnee] -> Selector4/1
  [RKneeStateOut] -> VAS muscle right/4
  HAM&HFL muscles right/3 -> Vector ConcatenateKnee/1
  Selector/1 -> GLU muscle right/1
  [RstanceOut] -> GAS muscle right/3
  [RphidphiAnkle] -> Selector7/1
  [RstanceOut] -> SOL&TA muscles right/2
  HAM&HFL muscles right/2 -> Vector ConcatenateHip/3
  Selector2/1 -> HAM&HFL muscles right/2
  [RphidphiAnkle] -> Selector6/1
  [RphidphiHip] -> Selector1/1
  [RstanceOut] -> VAS muscle right/5
  [RphidphiHip] -> Selector/1
  [RphidphiHip] -> HipJoint right/1
  [RphidphiKnee] -> Selector2/1
  HipJoint right/1 -> [RTauHip]
  KneeJoint right/1 -> [RTauKnee]
  AnkleJoint right/1 -> [RTauAnkle]
  [RdxThighOut] -> GLU muscle right/2
  [LonR] -> GLU muscle right/3
  [RstanceOut] -> GLU muscle right/4
  [RdxThighOut] -> HAM&HFL muscles right/3
  [LonR] -> HAM&HFL muscles right/4
  [RstanceOut] -> HAM&HFL muscles right/5
  RphidphiHip/1 -> [RphidphiHip]
  RphidphiKnee/1 -> [RphidphiKnee]
  RphidphiAnkle/1 -> [RphidphiAnkle]
  [RTauHip] -> RTauHip/1
  [RTauKnee] -> RTauKnee/1
  [RTauAnkle] -> RTauAnkle/1
  HipJoint right/2 -> [RHipStop]
  KneeJoint right/2 -> [RKneeStop]
  AnkleJoint right/2 -> [RAnkleStop]
  GLU muscle right/2 -> [REnergyGLU]
  HAM&HFL muscles right/4 -> [REnergyHFL]
  HAM&HFL muscles right/5 -> [REnergyHAM]
  VAS muscle right/2 -> [REnergyVAS]
  SOL&TA muscles right/3 -> [REnergyTA]
  SOL&TA muscles right/4 -> [REnergySOL]
  GAS muscle right/3 -> [REnergyGAS]

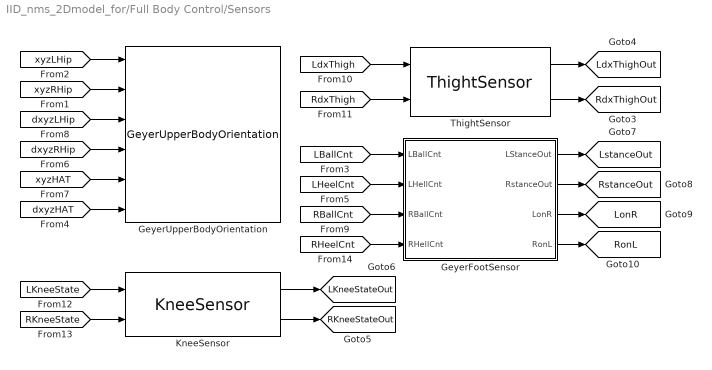
== system IID_nms_2Dmodel_for/Full Body Control/Sensors ==
  GeyerFootSensor : Subsystem  AncestorBlock=cpg_lib/GeyerFootSensor
  GeyerUpperBodyOrientation : cpg_lib/GeyerUpperBodyOrientation
  KneeSensor : cpg_lib/KneeSensor
  ThightSensor : cpg_lib/ThightSensor
  tag scope: LKneeStateOut=global, LdxThighOut=global, LonR=global, LstanceOut=global, RKneeStateOut=global, RdxThighOut=global, RonL=global, RstanceOut=global
  wires:
  [xyzLHip] -> GeyerUpperBodyOrientation/1
  ThightSensor/2 -> [RdxThighOut]
  [dxyzRHip] -> GeyerUpperBodyOrientation/4
  [dxyzHAT] -> GeyerUpperBodyOrientation/6
  [RdxThigh] -> ThightSensor/2
  ThightSensor/1 -> [LdxThighOut]
  [xyzRHip] -> GeyerUpperBodyOrientation/2
  [dxyzLHip] -> GeyerUpperBodyOrientation/3
  [xyzHAT] -> GeyerUpperBodyOrientation/5
  [LdxThigh] -> ThightSensor/1
  [LKneeState] -> KneeSensor/1
  [RKneeState] -> KneeSensor/2
  KneeSensor/1 -> [LKneeStateOut]
  KneeSensor/2 -> [RKneeStateOut]
  [LBallCnt] -> GeyerFootSensor/1(LBallCnt)
  [LHeelCnt] -> GeyerFootSensor/2(LHellCnt)
  [RBallCnt] -> GeyerFootSensor/3(RBallCnt)
  [RHeelCnt] -> GeyerFootSensor/4(RHellCnt)
  GeyerFootSensor/1(LStanceOut) -> [LstanceOut]
  GeyerFootSensor/2(RstanceOut) -> [RstanceOut]
  GeyerFootSensor/3(LonR) -> [LonR]
  GeyerFootSensor/4(RonL) -> [RonL]

== system IID_nms_2Dmodel_for/Body Mechanics Layer/Right Heel Contact/Ground Friction Model ==
  note: Vertical Ground Stiction Model
  note: Horizontal Ground Friction Model
  dy [m] : Inport
  vy [m/s] : Inport  Port=2
  x [m] : Inport  Port=3
  vx [m/s] : Inport  Port=4
  Contact! : EnablePort  StatesWhenEnabling=reset
  Data Type Conversion : DataTypeConversion  OutDataTypeStr=double
  Friction Switch : Subsystem
  Gain3 : Gain  Gain=k_gy
  Gain4 : Gain  Gain=1/v_gy_max
  Logical Operator : Logic  Operator=NOT  AllPortsSameDT=off  OutDataTypeStr=boolean
  Mux1 : Mux  Inputs=2
  Sum1 : Sum
  X-Axis Kinetic Friction Model : Subsystem
  X-Axis Static Friction Model : Subsystem
  Y-Axis Ground Force : Fcn  Expr="- u(1)  *  (1-u(2)) * (u(2)<1)"
  Fy_Ground[N] : Outport  OutputWhenDisabled=reset  InitialOutput=0
      settings: AttributesFormatString=initial = '%<InitialOutput>'\nwhen disabled = '%<OutputWhenDisabled>'
  Fx_Friction [N] : Outport  Port=2  OutputWhenDisabled=reset  InitialOutput=0
      settings: AttributesFormatString=initial = '%<InitialOutput>'\nwhen\ndisabled\n'%<OutputWhenDisabled>'
  Stiction! : Outport  Port=3  OutputWhenDisabled=reset  InitialOutput=0
      settings: AttributesFormatString=initial = '%<InitialOutput>'\nwhen\ndisabled\n'%<OutputWhenDisabled>'
  wires:
  Gain4/1 -> Mux1/2
  Gain3/1 -> Mux1/1
  Mux1/1 -> Y-Axis Ground Force/1
  Data Type Conversion/1 -> Stiction!/1
  Logical Operator/1 -> X-Axis Kinetic Friction Model/Enable
  X-Axis Kinetic Friction Model/2(Stiction!) -> Friction Switch/2(Stick!)
  X-Axis Static Friction Model/2(Sliding!) -> Friction Switch/1(Slide!)
  Friction Switch/1(Stiction) -> Data Type Conversion/1, Logical Operator/1, X-Axis Static Friction Model/Enable
  Sum1/1 -> Fx_Friction [N]/1
  X-Axis Static Friction Model/1(F_Stick [N]) -> Sum1/1
  X-Axis Kinetic Friction Model/3(F_Slide [N]) -> Sum1/2
  X-Axis Kinetic Friction Model/1(posFP [m]) -> X-Axis Static Friction Model/4(posFP [m])
  vx [m/s]/1 -> X-Axis Kinetic Friction Model/2(vel [m/s]), X-Axis Static Friction Model/3(vel [m/s])
  x [m]/1 -> X-Axis Kinetic Friction Model/1(pos [m]), X-Axis Static Friction Model/2(pos [m])
  vy [m/s]/1 -> Gain4/1
  dy [m]/1 -> Gain3/1
  Y-Axis Ground Force/1 -> Fy_Ground[N]/1, X-Axis Kinetic Friction Model/3(F_Normal [N]), X-Axis Static Friction Model/1(F_Normal [N])

== system IID_nms_2Dmodel_for/Body Mechanics Layer/Right Heel Contact1/Ground Friction Model ==
  note: Horizontal Ground Friction Model
  note: Vertical Ground Stiction Model
  dy [m] : Inport
  vy [m/s] : Inport  Port=2
  x [m] : Inport  Port=3
  vx [m/s] : Inport  Port=4
  Contact! : EnablePort  StatesWhenEnabling=reset
  Data Type Conversion : DataTypeConversion  OutDataTypeStr=double
  Friction Switch : Subsystem
  Gain3 : Gain  Gain=k_gy
  Gain4 : Gain  Gain=1/v_gy_max
  Logical Operator : Logic  Operator=NOT  AllPortsSameDT=off  OutDataTypeStr=boolean
  Mux1 : Mux  Inputs=2
  Sum1 : Sum
  X-Axis Kinetic Friction Model : Subsystem
  X-Axis Static Friction Model : Subsystem
  Y-Axis Ground Force : Fcn  Expr="- u(1)  *  (1-u(2)) * (u(2)<1)"
  Fy_Ground[N] : Outport  OutputWhenDisabled=reset  InitialOutput=0
      settings: AttributesFormatString=initial = '%<InitialOutput>'\nwhen disabled = '%<OutputWhenDisabled>'
  Fx_Friction [N] : Outport  Port=2  OutputWhenDisabled=reset  InitialOutput=0
      settings: AttributesFormatString=initial = '%<InitialOutput>'\nwhen\ndisabled\n'%<OutputWhenDisabled>'
  Stiction! : Outport  Port=3  OutputWhenDisabled=reset  InitialOutput=0
      settings: AttributesFormatString=initial = '%<InitialOutput>'\nwhen\ndisabled\n'%<OutputWhenDisabled>'
  wires:
  Y-Axis Ground Force/1 -> X-Axis Static Friction Model/1(F_Normal [N]), X-Axis Kinetic Friction Model/3(F_Normal [N]), Fy_Ground[N]/1
  dy [m]/1 -> Gain3/1
  vy [m/s]/1 -> Gain4/1
  x [m]/1 -> X-Axis Static Friction Model/2(pos [m]), X-Axis Kinetic Friction Model/1(pos [m])
  vx [m/s]/1 -> X-Axis Static Friction Model/3(vel [m/s]), X-Axis Kinetic Friction Model/2(vel [m/s])
  X-Axis Kinetic Friction Model/1(posFP [m]) -> X-Axis Static Friction Model/4(posFP [m])
  X-Axis Kinetic Friction Model/3(F_Slide [N]) -> Sum1/2
  X-Axis Static Friction Model/1(F_Stick [N]) -> Sum1/1
  Sum1/1 -> Fx_Friction [N]/1
  Friction Switch/1(Stiction) -> X-Axis Static Friction Model/Enable, Logical Operator/1, Data Type Conversion/1
  X-Axis Static Friction Model/2(Sliding!) -> Friction Switch/1(Slide!)
  X-Axis Kinetic Friction Model/2(Stiction!) -> Friction Switch/2(Stick!)
  Logical Operator/1 -> X-Axis Kinetic Friction Model/Enable
  Data Type Conversion/1 -> Stiction!/1
  Mux1/1 -> Y-Axis Ground Force/1
  Gain3/1 -> Mux1/1
  Gain4/1 -> Mux1/2

== system IID_nms_2Dmodel_for/Body Mechanics Layer/Right Heel Contact2/Ground Friction Model ==
  note: Vertical Ground Stiction Model
  note: Horizontal Ground Friction Model
  dy [m] : Inport
  vy [m/s] : Inport  Port=2
  x [m] : Inport  Port=3
  vx [m/s] : Inport  Port=4
  Contact! : EnablePort  StatesWhenEnabling=reset
  Data Type Conversion : DataTypeConversion  OutDataTypeStr=double
  Friction Switch : Subsystem
  Gain3 : Gain  Gain=k_gy
  Gain4 : Gain  Gain=1/v_gy_max
  Logical Operator : Logic  Operator=NOT  AllPortsSameDT=off  OutDataTypeStr=boolean
  Mux1 : Mux  Inputs=2
  Sum1 : Sum
  X-Axis Kinetic Friction Model : Subsystem
  X-Axis Static Friction Model : Subsystem
  Y-Axis Ground Force : Fcn  Expr="- u(1)  *  (1-u(2)) * (u(2)<1)"
  Fy_Ground[N] : Outport  OutputWhenDisabled=reset  InitialOutput=0
      settings: AttributesFormatString=initial = '%<InitialOutput>'\nwhen disabled = '%<OutputWhenDisabled>'
  Fx_Friction [N] : Outport  Port=2  OutputWhenDisabled=reset  InitialOutput=0
      settings: AttributesFormatString=initial = '%<InitialOutput>'\nwhen\ndisabled\n'%<OutputWhenDisabled>'
  Stiction! : Outport  Port=3  OutputWhenDisabled=reset  InitialOutput=0
      settings: AttributesFormatString=initial = '%<InitialOutput>'\nwhen\ndisabled\n'%<OutputWhenDisabled>'
  wires:
  Gain4/1 -> Mux1/2
  Gain3/1 -> Mux1/1
  Mux1/1 -> Y-Axis Ground Force/1
  Data Type Conversion/1 -> Stiction!/1
  Logical Operator/1 -> X-Axis Kinetic Friction Model/Enable
  X-Axis Kinetic Friction Model/2(Stiction!) -> Friction Switch/2(Stick!)
  X-Axis Static Friction Model/2(Sliding!) -> Friction Switch/1(Slide!)
  Friction Switch/1(Stiction) -> Data Type Conversion/1, Logical Operator/1, X-Axis Static Friction Model/Enable
  Sum1/1 -> Fx_Friction [N]/1
  X-Axis Static Friction Model/1(F_Stick [N]) -> Sum1/1
  X-Axis Kinetic Friction Model/3(F_Slide [N]) -> Sum1/2
  X-Axis Kinetic Friction Model/1(posFP [m]) -> X-Axis Static Friction Model/4(posFP [m])
  vx [m/s]/1 -> X-Axis Kinetic Friction Model/2(vel [m/s]), X-Axis Static Friction Model/3(vel [m/s])
  x [m]/1 -> X-Axis Kinetic Friction Model/1(pos [m]), X-Axis Static Friction Model/2(pos [m])
  vy [m/s]/1 -> Gain4/1
  dy [m]/1 -> Gain3/1
  Y-Axis Ground Force/1 -> Fy_Ground[N]/1, X-Axis Kinetic Friction Model/3(F_Normal [N]), X-Axis Static Friction Model/1(F_Normal [N])
